simulink model "SG_SetMotorValueToZero"  (R2022a)
settings: Solver=ode4  StartTime=0.0  StopTime=inf  FixedStep=1/1000  RelTol=1e-3
libraries: speedgoatlib_IO691 x9, canmsglib x8
settings Model: SimulationMode=external  ExtModeEnableFloating=off  Creator=Mechatronics  LastModifiedBy=Mechatronics
settings SolverCC: ConcurrentTasks=on  AlgebraicLoopSolver=TrustRegion  PositivePriorityOrder=on
settings OptimizationCC: BlockReduction=off  OptimizeBlockIOStorage=off
settings DebuggingCC: TasksWithSamePriorityMsg=none  UnconnectedInputMsg=warning  UnconnectedOutputMsg=warning  UnconnectedLineMsg=warning  SFMachineParentedDataDiag=warning
settings HardwareCC: ProdBitPerLong=64  ProdLongLongMode=on  ProdHWDeviceType=Intel->x86-64 (Linux 64)
settings RTWCC: Description=Simulink Real-Time  SystemTargetFile=slrealtime.tlc  TemplateMakefile=slrealtime_default_tmf  Toolchain=Simulink Real-Time Toolchain  BuildConfiguration=Faster Runs  CodeExecutionProfiling=on  TargetLang=C++  DLArmComputeVersion=19.05
settings SimulinkRealTimeTargetCC: UseGCCFastMath=on

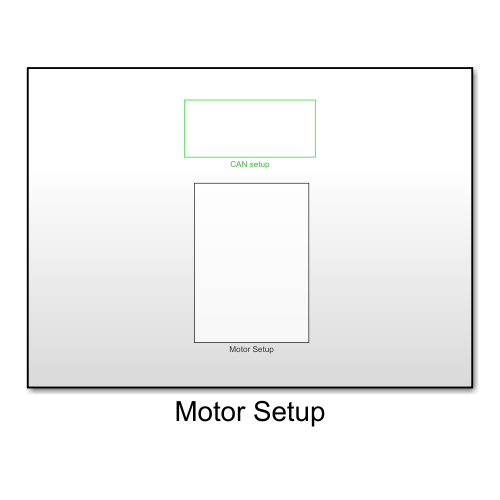
[thumbnail: Simulink's stored preview of the top-level diagram]
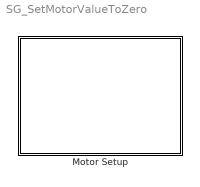
== system SG_SetMotorValueToZero ==
  Motor Setup : Subsystem

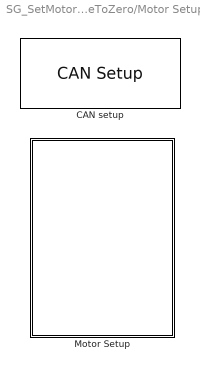
== system SG_SetMotorValueToZero/Motor Setup ==
  CAN setup : speedgoatlib_IO691/Legacy/CAN Setup   moduletype=IO691  id=1  pciSlot=-1  chn1=CAN (HS)  chn2=CAN (HS)  chn3=Disabled  chn4=Disabled  initStruct=[]  termStruct=[struct('Channel',1,'Protocol','CAN','BRS',0,'Type','Standard','Identifier',3,'Data',[255, 255, 255, 255, 255, 255, 255, 253],'Pause',0.001),struct('Channel',1,'Protocol','CAN','BRS',0,'Type','Standard','Identifier',2,'Data',[255, 255, 255, 255, 255, 255, 255, 253],'Pause',0.001),struct('Channel',2,'Protocol','CAN','BRS',0,'Type','Standard','Identifier',4,'Data',[255, 255, 255, 255, 255, 255, 255, 253],'Pause',0.001), struct('Channel',2,'Protocol','CAN','BRS',0,'Type','Standard','Identifier',1,'Data',[255, 255, 255, 255, 255, 255, 255, 253],'Pause',0.001)]  ArbitrationbdrChn1=1.0 MBaud  ArbitrationManbdrChn1=[2,8,31,8]  FdbdrChn1=1.0 MBaud  FdManbdrChn1=[2,8,31,8]  ArbitrationbdrChn2=1.0 MBaud  ArbitrationManbdrChn2=[2,8,31,8]  FdbdrChn2=1.0 MBaud  FdManbdrChn2=[2,8,31,8]  ArbitrationbdrChn3=1.0 MBaud  ArbitrationManbdrChn3=[2,8,31,8]  FdbdrChn3=5.0 MBaud  FdManbdrChn3=[2,2,5,2]  ArbitrationbdrChn4=1.0 MBaud  ArbitrationManbdrChn4=[2,8,31,8]  FdbdrChn4=5.0 MBaud  FdManbdrChn4=[2,2,5,2]  moduleInitValues=[691 1 -1 -1]
      settings: SourceProductName=Simulink Real-Time: Speedgoat I/O Blockset
  Motor Setup : Subsystem

== system SG_SetMotorValueToZero/Motor Setup/Motor Setup ==
  Back : Subsystem
  Front : Subsystem

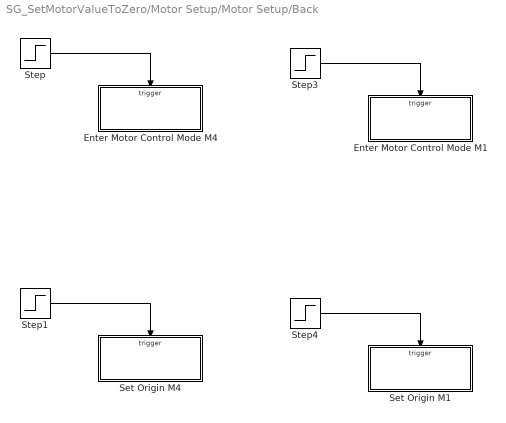
== system SG_SetMotorValueToZero/Motor Setup/Motor Setup/Back ==
  Enter Motor Control Mode M1 : Subsystem  TreatAsAtomicUnit=on
  Enter Motor Control Mode M4 : Subsystem  TreatAsAtomicUnit=on
  Set Origin M1 : Subsystem  TreatAsAtomicUnit=on
  Set Origin M4 : Subsystem  TreatAsAtomicUnit=on
  Step : Step  Time=3
  Step1 : Step  Time=2.5
  Step3 : Step  Time=4
  Step4 : Step  Time=3.5
  wires:
  Step1/1 -> Set Origin M4/Trigger
  Step4/1 -> Set Origin M1/Trigger
  Step/1 -> Enter Motor Control Mode M4/Trigger
  Step3/1 -> Enter Motor Control Mode M1/Trigger

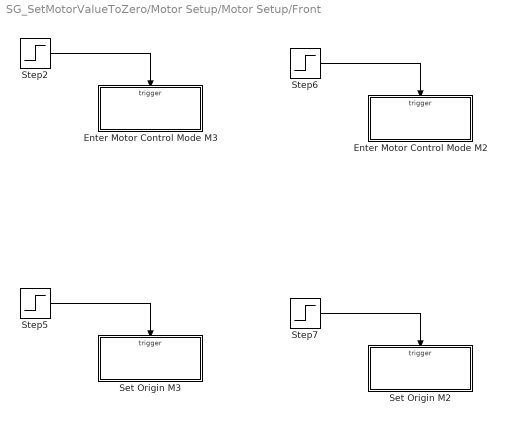
== system SG_SetMotorValueToZero/Motor Setup/Motor Setup/Front ==
  Enter Motor Control Mode M2 : Subsystem  TreatAsAtomicUnit=on
  Enter Motor Control Mode M3 : Subsystem  TreatAsAtomicUnit=on
  Set Origin M2 : Subsystem  TreatAsAtomicUnit=on
  Set Origin M3 : Subsystem  TreatAsAtomicUnit=on
  Step2 : Step  Time=1.0
  Step5 : Step  Time=0.5
  Step6 : Step  Time=2
  Step7 : Step  Time=1.5
  wires:
  Step5/1 -> Set Origin M3/Trigger
  Step7/1 -> Set Origin M2/Trigger
  Step2/1 -> Enter Motor Control Mode M3/Trigger
  Step6/1 -> Enter Motor Control Mode M2/Trigger

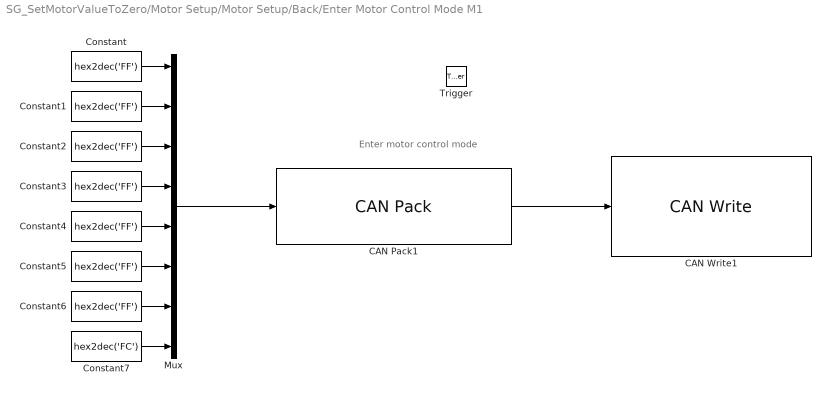
== system SG_SetMotorValueToZero/Motor Setup/Motor Setup/Back/Enter Motor Control Mode M1 ==
  note: Enter motor control mode
  Trigger : TriggerPort  VariantControl=Variant
  CAN Pack1 : canmsglib/CAN Pack  MsgList=(none)  MsgName=CAN Msg  MsgIDType=Standard (11-bit identifier)  MsgIdentifier=1  MsgLength=8  Remote=off  ApplyMinMax=off  BusOutput=off  SignalInfo={ 'Motor postition 8-H', '0', '8', 'LE', 'unsigned', 'Standard', '0', '1', '0', '-Inf', 'Inf'; 'Motor position 8-L', '8', '8', 'LE', 'unsigned', 'Standard', '0', '1', '0', '-Inf', 'Inf'; 'Motor seed 8-H', '16', '8', 'LE', 'unsigned', 'Standard', '0', '1', '0', '-Inf', 'Inf'; 'Motor speed 4-L', '28', '4', 'LE', 'unsigned', 'Standard', '0', '1', '0', '-Inf', 'Inf'; 'KP 4-H', '24', '4', 'LE', 'unsigned', 'Standard', '0', '1', '0', '-Inf', 'Inf'; 'KP 8-L', '32', '8', 'LE', 'unsigned', 'Standard', '0', '1', '0', '-Inf', 'Inf'; 'KP 8-H', '40', '8', 'LE', 'unsigned', 'Standard', '0', '1', '0', '-Inf', 'Inf'; 'KD 4-L', '52', '4', 'LE', 'unsigned', 'Standard', '0', '1', '0', '-Inf', 'Inf'; 'Current 4-H', '48', '4', 'LE', 'unsigned', 'Standard', '0', '1', '0', '-Inf', 'Inf'; 'Current 8-L', '56', '8', 'LE', 'unsigned', 'Standard', '0', '1', '0', '-Inf', 'Inf' }
      settings: SourceProductBaseCode=XP,ME,VN  DataFormat=raw data
  CAN Write1 : speedgoatlib_IO691/Legacy/CAN Write  id=1  ts=-1  channel=2  messageType=CAN  BusInput=off  enableStatusPort=off  canType=CAN (HS)  initValues=[691 1 -1 1 1 1 0 0]
      settings: SourceProductName=Simulink Real-Time: Speedgoat Library
  Constant{,1..6} (7 alike) : Constant  Value=hex2dec('FF')  OutDataTypeStr=uint8  SampleTime=-1
  Constant7 : Constant  Value=hex2dec('FC')  OutDataTypeStr=uint8  SampleTime=-1
  Mux : Mux  Inputs=8
  wires:
  CAN Pack1/1 -> CAN Write1/1
  Mux/1 -> CAN Pack1/1
  Constant7/1 -> Mux/8
  Constant4/1 -> Mux/5
  Constant1/1 -> Mux/2
  Constant5/1 -> Mux/6
  Constant3/1 -> Mux/4
  Constant2/1 -> Mux/3
  Constant/1 -> Mux/1
  Constant6/1 -> Mux/7

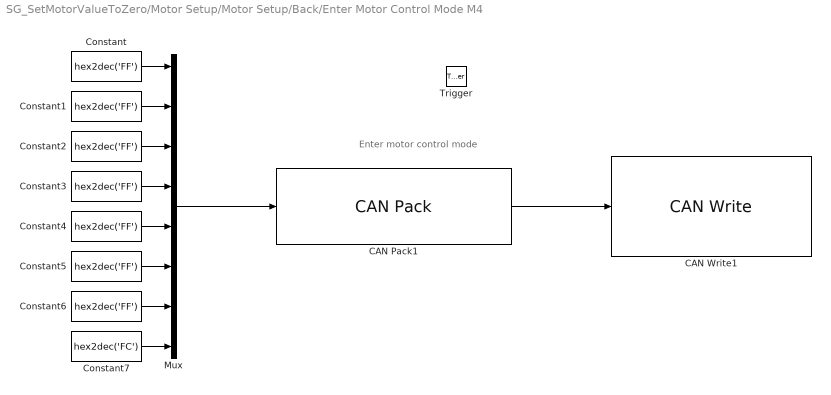
== system SG_SetMotorValueToZero/Motor Setup/Motor Setup/Back/Enter Motor Control Mode M4 ==
  note: Enter motor control mode
  Trigger : TriggerPort  VariantControl=Variant
  CAN Pack1 : canmsglib/CAN Pack  MsgList=(none)  MsgName=CAN Msg  MsgIDType=Standard (11-bit identifier)  MsgIdentifier=4  MsgLength=8  Remote=off  ApplyMinMax=off  BusOutput=off  SignalInfo={ 'Motor postition 8-H', '0', '8', 'LE', 'unsigned', 'Standard', '0', '1', '0', '-Inf', 'Inf'; 'Motor position 8-L', '8', '8', 'LE', 'unsigned', 'Standard', '0', '1', '0', '-Inf', 'Inf'; 'Motor seed 8-H', '16', '8', 'LE', 'unsigned', 'Standard', '0', '1', '0', '-Inf', 'Inf'; 'Motor speed 4-L', '28', '4', 'LE', 'unsigned', 'Standard', '0', '1', '0', '-Inf', 'Inf'; 'KP 4-H', '24', '4', 'LE', 'unsigned', 'Standard', '0', '1', '0', '-Inf', 'Inf'; 'KP 8-L', '32', '8', 'LE', 'unsigned', 'Standard', '0', '1', '0', '-Inf', 'Inf'; 'KP 8-H', '40', '8', 'LE', 'unsigned', 'Standard', '0', '1', '0', '-Inf', 'Inf'; 'KD 4-L', '52', '4', 'LE', 'unsigned', 'Standard', '0', '1', '0', '-Inf', 'Inf'; 'Current 4-H', '48', '4', 'LE', 'unsigned', 'Standard', '0', '1', '0', '-Inf', 'Inf'; 'Current 8-L', '56', '8', 'LE', 'unsigned', 'Standard', '0', '1', '0', '-Inf', 'Inf' }
      settings: SourceProductBaseCode=XP,ME,VN  DataFormat=raw data
  CAN Write1 : speedgoatlib_IO691/Legacy/CAN Write  id=1  ts=-1  channel=2  messageType=CAN  BusInput=off  enableStatusPort=off  canType=CAN (HS)  initValues=[691 1 -1 1 1 1 0 0]
      settings: SourceProductName=Simulink Real-Time: Speedgoat Library
  Constant{,1..6} (7 alike) : Constant  Value=hex2dec('FF')  OutDataTypeStr=uint8  SampleTime=-1
  Constant7 : Constant  Value=hex2dec('FC')  OutDataTypeStr=uint8  SampleTime=-1
  Mux : Mux  Inputs=8
  wires:
  CAN Pack1/1 -> CAN Write1/1
  Mux/1 -> CAN Pack1/1
  Constant7/1 -> Mux/8
  Constant4/1 -> Mux/5
  Constant1/1 -> Mux/2
  Constant5/1 -> Mux/6
  Constant3/1 -> Mux/4
  Constant2/1 -> Mux/3
  Constant/1 -> Mux/1
  Constant6/1 -> Mux/7

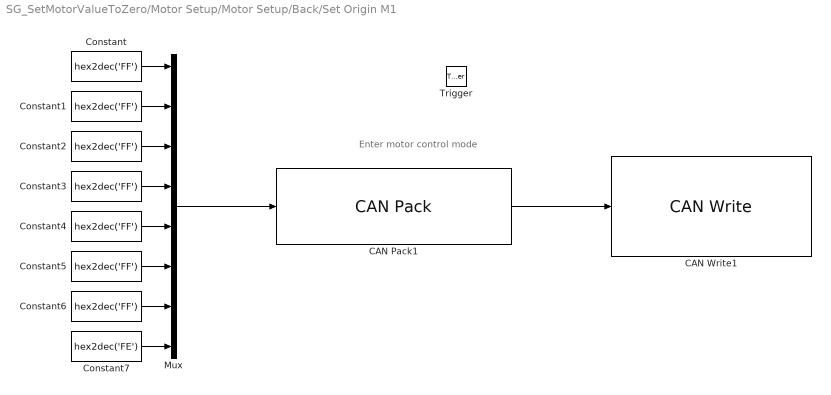
== system SG_SetMotorValueToZero/Motor Setup/Motor Setup/Back/Set Origin M1 ==
  note: Enter motor control mode
  Trigger : TriggerPort  VariantControl=Variant
  CAN Pack1 : canmsglib/CAN Pack  MsgList=(none)  MsgName=CAN Msg  MsgIDType=Standard (11-bit identifier)  MsgIdentifier=1  MsgLength=8  Remote=off  ApplyMinMax=off  BusOutput=off  SignalInfo={ 'Motor postition 8-H', '0', '8', 'LE', 'unsigned', 'Standard', '0', '1', '0', '-Inf', 'Inf'; 'Motor position 8-L', '8', '8', 'LE', 'unsigned', 'Standard', '0', '1', '0', '-Inf', 'Inf'; 'Motor seed 8-H', '16', '8', 'LE', 'unsigned', 'Standard', '0', '1', '0', '-Inf', 'Inf'; 'Motor speed 4-L', '28', '4', 'LE', 'unsigned', 'Standard', '0', '1', '0', '-Inf', 'Inf'; 'KP 4-H', '24', '4', 'LE', 'unsigned', 'Standard', '0', '1', '0', '-Inf', 'Inf'; 'KP 8-L', '32', '8', 'LE', 'unsigned', 'Standard', '0', '1', '0', '-Inf', 'Inf'; 'KP 8-H', '40', '8', 'LE', 'unsigned', 'Standard', '0', '1', '0', '-Inf', 'Inf'; 'KD 4-L', '52', '4', 'LE', 'unsigned', 'Standard', '0', '1', '0', '-Inf', 'Inf'; 'Current 4-H', '48', '4', 'LE', 'unsigned', 'Standard', '0', '1', '0', '-Inf', 'Inf'; 'Current 8-L', '56', '8', 'LE', 'unsigned', 'Standard', '0', '1', '0', '-Inf', 'Inf' }
      settings: SourceProductBaseCode=XP,ME,VN  DataFormat=raw data
  CAN Write1 : speedgoatlib_IO691/Legacy/CAN Write  id=1  ts=-1  channel=2  messageType=CAN  BusInput=off  enableStatusPort=off  canType=CAN (HS)  initValues=[691 1 -1 1 1 1 0 0]
      settings: SourceProductName=Simulink Real-Time: Speedgoat Library
  Constant{,1..6} (7 alike) : Constant  Value=hex2dec('FF')  OutDataTypeStr=uint8  SampleTime=-1
  Constant7 : Constant  Value=hex2dec('FE')  OutDataTypeStr=uint8  SampleTime=-1
  Mux : Mux  Inputs=8
  wires:
  CAN Pack1/1 -> CAN Write1/1
  Mux/1 -> CAN Pack1/1
  Constant7/1 -> Mux/8
  Constant4/1 -> Mux/5
  Constant1/1 -> Mux/2
  Constant5/1 -> Mux/6
  Constant3/1 -> Mux/4
  Constant2/1 -> Mux/3
  Constant/1 -> Mux/1
  Constant6/1 -> Mux/7

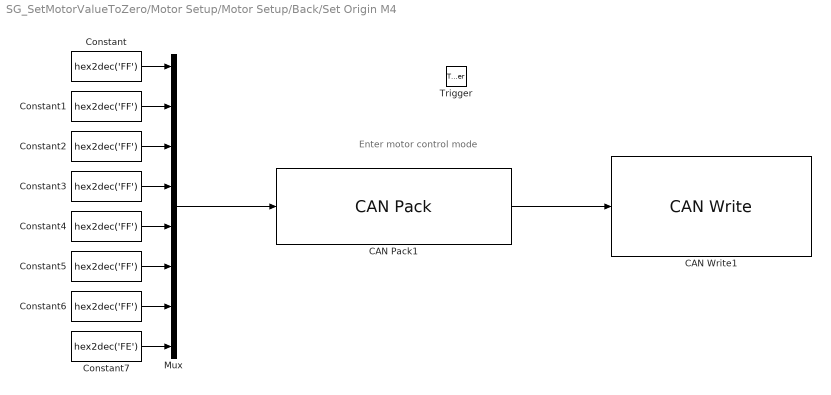
== system SG_SetMotorValueToZero/Motor Setup/Motor Setup/Back/Set Origin M4 ==
  note: Enter motor control mode
  Trigger : TriggerPort  VariantControl=Variant
  CAN Pack1 : canmsglib/CAN Pack  MsgList=(none)  MsgName=CAN Msg  MsgIDType=Standard (11-bit identifier)  MsgIdentifier=4  MsgLength=8  Remote=off  ApplyMinMax=off  BusOutput=off  SignalInfo={ 'Motor postition 8-H', '0', '8', 'LE', 'unsigned', 'Standard', '0', '1', '0', '-Inf', 'Inf'; 'Motor position 8-L', '8', '8', 'LE', 'unsigned', 'Standard', '0', '1', '0', '-Inf', 'Inf'; 'Motor seed 8-H', '16', '8', 'LE', 'unsigned', 'Standard', '0', '1', '0', '-Inf', 'Inf'; 'Motor speed 4-L', '28', '4', 'LE', 'unsigned', 'Standard', '0', '1', '0', '-Inf', 'Inf'; 'KP 4-H', '24', '4', 'LE', 'unsigned', 'Standard', '0', '1', '0', '-Inf', 'Inf'; 'KP 8-L', '32', '8', 'LE', 'unsigned', 'Standard', '0', '1', '0', '-Inf', 'Inf'; 'KP 8-H', '40', '8', 'LE', 'unsigned', 'Standard', '0', '1', '0', '-Inf', 'Inf'; 'KD 4-L', '52', '4', 'LE', 'unsigned', 'Standard', '0', '1', '0', '-Inf', 'Inf'; 'Current 4-H', '48', '4', 'LE', 'unsigned', 'Standard', '0', '1', '0', '-Inf', 'Inf'; 'Current 8-L', '56', '8', 'LE', 'unsigned', 'Standard', '0', '1', '0', '-Inf', 'Inf' }
      settings: SourceProductBaseCode=XP,ME,VN  DataFormat=raw data
  CAN Write1 : speedgoatlib_IO691/Legacy/CAN Write  id=1  ts=-1  channel=2  messageType=CAN  BusInput=off  enableStatusPort=off  canType=CAN (HS)  initValues=[691 1 -1 1 1 1 0 0]
      settings: SourceProductName=Simulink Real-Time: Speedgoat Library
  Constant{,1..6} (7 alike) : Constant  Value=hex2dec('FF')  OutDataTypeStr=uint8  SampleTime=-1
  Constant7 : Constant  Value=hex2dec('FE')  OutDataTypeStr=uint8  SampleTime=-1
  Mux : Mux  Inputs=8
  wires:
  CAN Pack1/1 -> CAN Write1/1
  Mux/1 -> CAN Pack1/1
  Constant7/1 -> Mux/8
  Constant4/1 -> Mux/5
  Constant1/1 -> Mux/2
  Constant5/1 -> Mux/6
  Constant3/1 -> Mux/4
  Constant2/1 -> Mux/3
  Constant/1 -> Mux/1
  Constant6/1 -> Mux/7

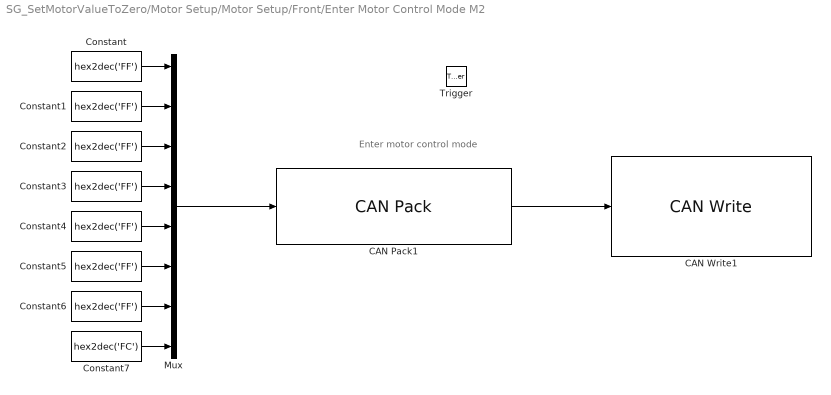
== system SG_SetMotorValueToZero/Motor Setup/Motor Setup/Front/Enter Motor Control Mode M2 ==
  note: Enter motor control mode
  Trigger : TriggerPort  VariantControl=Variant
  CAN Pack1 : canmsglib/CAN Pack  MsgList=(none)  MsgName=CAN Msg  MsgIDType=Standard (11-bit identifier)  MsgIdentifier=2  MsgLength=8  Remote=off  ApplyMinMax=off  BusOutput=off  SignalInfo={ 'Motor postition 8-H', '0', '8', 'LE', 'unsigned', 'Standard', '0', '1', '0', '-Inf', 'Inf'; 'Motor position 8-L', '8', '8', 'LE', 'unsigned', 'Standard', '0', '1', '0', '-Inf', 'Inf'; 'Motor seed 8-H', '16', '8', 'LE', 'unsigned', 'Standard', '0', '1', '0', '-Inf', 'Inf'; 'Motor speed 4-L', '28', '4', 'LE', 'unsigned', 'Standard', '0', '1', '0', '-Inf', 'Inf'; 'KP 4-H', '24', '4', 'LE', 'unsigned', 'Standard', '0', '1', '0', '-Inf', 'Inf'; 'KP 8-L', '32', '8', 'LE', 'unsigned', 'Standard', '0', '1', '0', '-Inf', 'Inf'; 'KP 8-H', '40', '8', 'LE', 'unsigned', 'Standard', '0', '1', '0', '-Inf', 'Inf'; 'KD 4-L', '52', '4', 'LE', 'unsigned', 'Standard', '0', '1', '0', '-Inf', 'Inf'; 'Current 4-H', '48', '4', 'LE', 'unsigned', 'Standard', '0', '1', '0', '-Inf', 'Inf'; 'Current 8-L', '56', '8', 'LE', 'unsigned', 'Standard', '0', '1', '0', '-Inf', 'Inf' }
      settings: SourceProductBaseCode=XP,ME,VN  DataFormat=raw data
  CAN Write1 : speedgoatlib_IO691/Legacy/CAN Write  id=1  ts=-1  channel=1  messageType=CAN  BusInput=off  enableStatusPort=off  canType=CAN (HS)  initValues=[691 1 -1 0 1 1 0 0]
      settings: SourceProductName=Simulink Real-Time: Speedgoat Library
  Constant{,1..6} (7 alike) : Constant  Value=hex2dec('FF')  OutDataTypeStr=uint8  SampleTime=-1
  Constant7 : Constant  Value=hex2dec('FC')  OutDataTypeStr=uint8  SampleTime=-1
  Mux : Mux  Inputs=8
  wires:
  CAN Pack1/1 -> CAN Write1/1
  Mux/1 -> CAN Pack1/1
  Constant7/1 -> Mux/8
  Constant4/1 -> Mux/5
  Constant1/1 -> Mux/2
  Constant5/1 -> Mux/6
  Constant3/1 -> Mux/4
  Constant2/1 -> Mux/3
  Constant/1 -> Mux/1
  Constant6/1 -> Mux/7

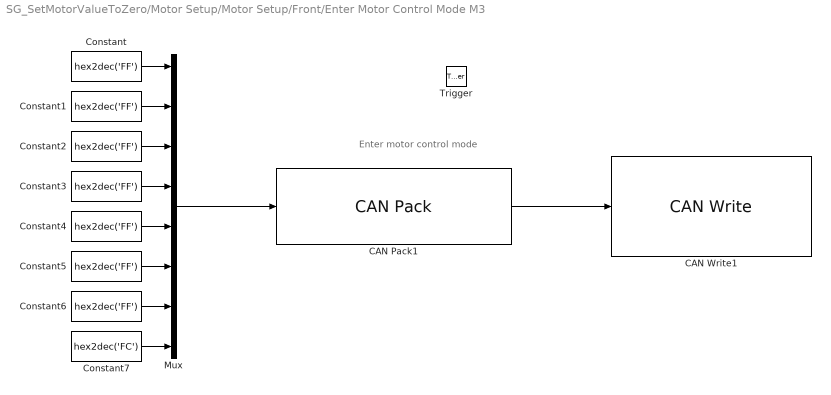
== system SG_SetMotorValueToZero/Motor Setup/Motor Setup/Front/Enter Motor Control Mode M3 ==
  note: Enter motor control mode
  Trigger : TriggerPort  VariantControl=Variant
  CAN Pack1 : canmsglib/CAN Pack  MsgList=(none)  MsgName=CAN Msg  MsgIDType=Standard (11-bit identifier)  MsgIdentifier=3  MsgLength=8  Remote=off  ApplyMinMax=off  BusOutput=off  SignalInfo={ 'Motor postition 8-H', '0', '8', 'LE', 'unsigned', 'Standard', '0', '1', '0', '-Inf', 'Inf'; 'Motor position 8-L', '8', '8', 'LE', 'unsigned', 'Standard', '0', '1', '0', '-Inf', 'Inf'; 'Motor seed 8-H', '16', '8', 'LE', 'unsigned', 'Standard', '0', '1', '0', '-Inf', 'Inf'; 'Motor speed 4-L', '28', '4', 'LE', 'unsigned', 'Standard', '0', '1', '0', '-Inf', 'Inf'; 'KP 4-H', '24', '4', 'LE', 'unsigned', 'Standard', '0', '1', '0', '-Inf', 'Inf'; 'KP 8-L', '32', '8', 'LE', 'unsigned', 'Standard', '0', '1', '0', '-Inf', 'Inf'; 'KP 8-H', '40', '8', 'LE', 'unsigned', 'Standard', '0', '1', '0', '-Inf', 'Inf'; 'KD 4-L', '52', '4', 'LE', 'unsigned', 'Standard', '0', '1', '0', '-Inf', 'Inf'; 'Current 4-H', '48', '4', 'LE', 'unsigned', 'Standard', '0', '1', '0', '-Inf', 'Inf'; 'Current 8-L', '56', '8', 'LE', 'unsigned', 'Standard', '0', '1', '0', '-Inf', 'Inf' }
      settings: SourceProductBaseCode=XP,ME,VN  DataFormat=raw data
  CAN Write1 : speedgoatlib_IO691/Legacy/CAN Write  id=1  ts=-1  channel=1  messageType=CAN  BusInput=off  enableStatusPort=off  canType=CAN (HS)  initValues=[691 1 -1 0 1 1 0 0]
      settings: SourceProductName=Simulink Real-Time: Speedgoat Library
  Constant{,1..6} (7 alike) : Constant  Value=hex2dec('FF')  OutDataTypeStr=uint8  SampleTime=-1
  Constant7 : Constant  Value=hex2dec('FC')  OutDataTypeStr=uint8  SampleTime=-1
  Mux : Mux  Inputs=8
  wires:
  CAN Pack1/1 -> CAN Write1/1
  Mux/1 -> CAN Pack1/1
  Constant7/1 -> Mux/8
  Constant4/1 -> Mux/5
  Constant1/1 -> Mux/2
  Constant5/1 -> Mux/6
  Constant3/1 -> Mux/4
  Constant2/1 -> Mux/3
  Constant/1 -> Mux/1
  Constant6/1 -> Mux/7

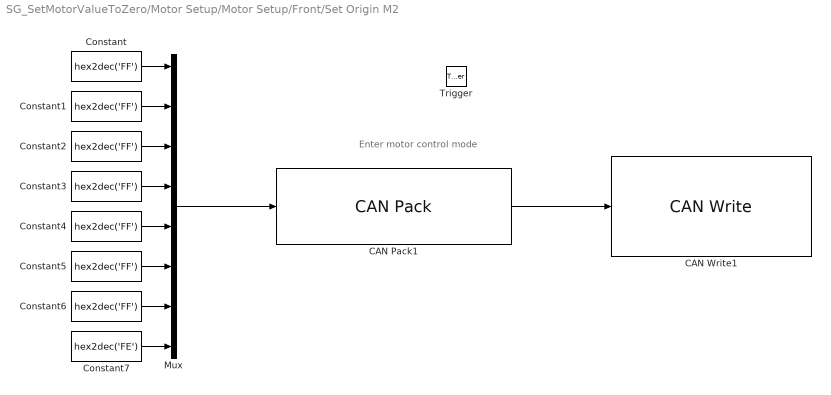
== system SG_SetMotorValueToZero/Motor Setup/Motor Setup/Front/Set Origin M2 ==
  note: Enter motor control mode
  Trigger : TriggerPort  VariantControl=Variant
  CAN Pack1 : canmsglib/CAN Pack  MsgList=(none)  MsgName=CAN Msg  MsgIDType=Standard (11-bit identifier)  MsgIdentifier=2  MsgLength=8  Remote=off  ApplyMinMax=off  BusOutput=off  SignalInfo={ 'Motor postition 8-H', '0', '8', 'LE', 'unsigned', 'Standard', '0', '1', '0', '-Inf', 'Inf'; 'Motor position 8-L', '8', '8', 'LE', 'unsigned', 'Standard', '0', '1', '0', '-Inf', 'Inf'; 'Motor seed 8-H', '16', '8', 'LE', 'unsigned', 'Standard', '0', '1', '0', '-Inf', 'Inf'; 'Motor speed 4-L', '28', '4', 'LE', 'unsigned', 'Standard', '0', '1', '0', '-Inf', 'Inf'; 'KP 4-H', '24', '4', 'LE', 'unsigned', 'Standard', '0', '1', '0', '-Inf', 'Inf'; 'KP 8-L', '32', '8', 'LE', 'unsigned', 'Standard', '0', '1', '0', '-Inf', 'Inf'; 'KP 8-H', '40', '8', 'LE', 'unsigned', 'Standard', '0', '1', '0', '-Inf', 'Inf'; 'KD 4-L', '52', '4', 'LE', 'unsigned', 'Standard', '0', '1', '0', '-Inf', 'Inf'; 'Current 4-H', '48', '4', 'LE', 'unsigned', 'Standard', '0', '1', '0', '-Inf', 'Inf'; 'Current 8-L', '56', '8', 'LE', 'unsigned', 'Standard', '0', '1', '0', '-Inf', 'Inf' }
      settings: SourceProductBaseCode=XP,ME,VN  DataFormat=raw data
  CAN Write1 : speedgoatlib_IO691/Legacy/CAN Write  id=1  ts=-1  channel=1  messageType=CAN  BusInput=off  enableStatusPort=off  canType=CAN (HS)  initValues=[691 1 -1 0 1 1 0 0]
      settings: SourceProductName=Simulink Real-Time: Speedgoat Library
  Constant{,1..6} (7 alike) : Constant  Value=hex2dec('FF')  OutDataTypeStr=uint8  SampleTime=-1
  Constant7 : Constant  Value=hex2dec('FE')  OutDataTypeStr=uint8  SampleTime=-1
  Mux : Mux  Inputs=8
  wires:
  CAN Pack1/1 -> CAN Write1/1
  Mux/1 -> CAN Pack1/1
  Constant7/1 -> Mux/8
  Constant4/1 -> Mux/5
  Constant1/1 -> Mux/2
  Constant5/1 -> Mux/6
  Constant3/1 -> Mux/4
  Constant2/1 -> Mux/3
  Constant/1 -> Mux/1
  Constant6/1 -> Mux/7

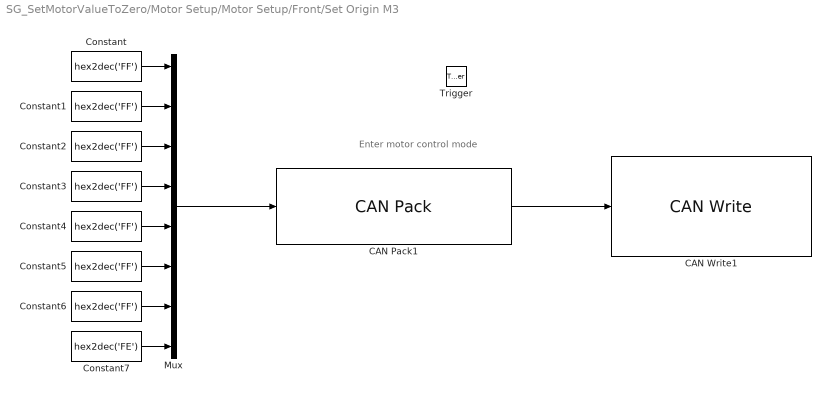
== system SG_SetMotorValueToZero/Motor Setup/Motor Setup/Front/Set Origin M3 ==
  note: Enter motor control mode
  Trigger : TriggerPort  VariantControl=Variant
  CAN Pack1 : canmsglib/CAN Pack  MsgList=(none)  MsgName=CAN Msg  MsgIDType=Standard (11-bit identifier)  MsgIdentifier=3  MsgLength=8  Remote=off  ApplyMinMax=off  BusOutput=off  SignalInfo={ 'Motor postition 8-H', '0', '8', 'LE', 'unsigned', 'Standard', '0', '1', '0', '-Inf', 'Inf'; 'Motor position 8-L', '8', '8', 'LE', 'unsigned', 'Standard', '0', '1', '0', '-Inf', 'Inf'; 'Motor seed 8-H', '16', '8', 'LE', 'unsigned', 'Standard', '0', '1', '0', '-Inf', 'Inf'; 'Motor speed 4-L', '28', '4', 'LE', 'unsigned', 'Standard', '0', '1', '0', '-Inf', 'Inf'; 'KP 4-H', '24', '4', 'LE', 'unsigned', 'Standard', '0', '1', '0', '-Inf', 'Inf'; 'KP 8-L', '32', '8', 'LE', 'unsigned', 'Standard', '0', '1', '0', '-Inf', 'Inf'; 'KP 8-H', '40', '8', 'LE', 'unsigned', 'Standard', '0', '1', '0', '-Inf', 'Inf'; 'KD 4-L', '52', '4', 'LE', 'unsigned', 'Standard', '0', '1', '0', '-Inf', 'Inf'; 'Current 4-H', '48', '4', 'LE', 'unsigned', 'Standard', '0', '1', '0', '-Inf', 'Inf'; 'Current 8-L', '56', '8', 'LE', 'unsigned', 'Standard', '0', '1', '0', '-Inf', 'Inf' }
      settings: SourceProductBaseCode=XP,ME,VN  DataFormat=raw data
  CAN Write1 : speedgoatlib_IO691/Legacy/CAN Write  id=1  ts=-1  channel=1  messageType=CAN  BusInput=off  enableStatusPort=off  canType=CAN (HS)  initValues=[691 1 -1 0 1 1 0 0]
      settings: SourceProductName=Simulink Real-Time: Speedgoat Library
  Constant{,1..6} (7 alike) : Constant  Value=hex2dec('FF')  OutDataTypeStr=uint8  SampleTime=-1
  Constant7 : Constant  Value=hex2dec('FE')  OutDataTypeStr=uint8  SampleTime=-1
  Mux : Mux  Inputs=8
  wires:
  CAN Pack1/1 -> CAN Write1/1
  Mux/1 -> CAN Pack1/1
  Constant7/1 -> Mux/8
  Constant4/1 -> Mux/5
  Constant1/1 -> Mux/2
  Constant5/1 -> Mux/6
  Constant3/1 -> Mux/4
  Constant2/1 -> Mux/3
  Constant/1 -> Mux/1
  Constant6/1 -> Mux/7
